simulink model "SPM_trial_2_simulink"  (R2022a)
settings: Solver=VariableStepAuto  StartTime=0.0  StopTime=500  RelTol=1e-3
values from neighbouring files (symbols this model uses):
  x_neg = 0:dx_n:del_n    [Generate_Amat_Electrolyte.m]
  x_pos = del_n+del_s:dx_p:del_n+del_s+del_p    [Generate_Amat_Electrolyte.m]
  x_sep = del_n:dx_s:del_n+del_s    [Generate_Amat_Electrolyte.m]
undefined symbols (not defined in the file or in its folder): CC, cs_init_n, cs_init_p, I, Iin, Ilim, Kaw, KI, nn, np, ns, sw, Vlim, Vmax
libraries: nesl_utility x6, fl_lib x4
settings Model: Creator=YASH PATHAK  LastModifiedBy=YASH PATHAK

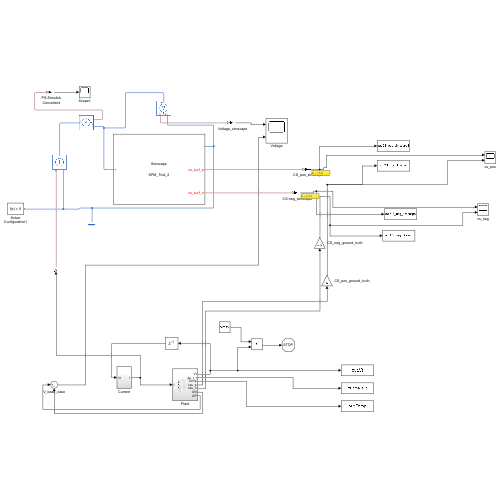
[thumbnail: Simulink's stored preview of the top-level diagram]
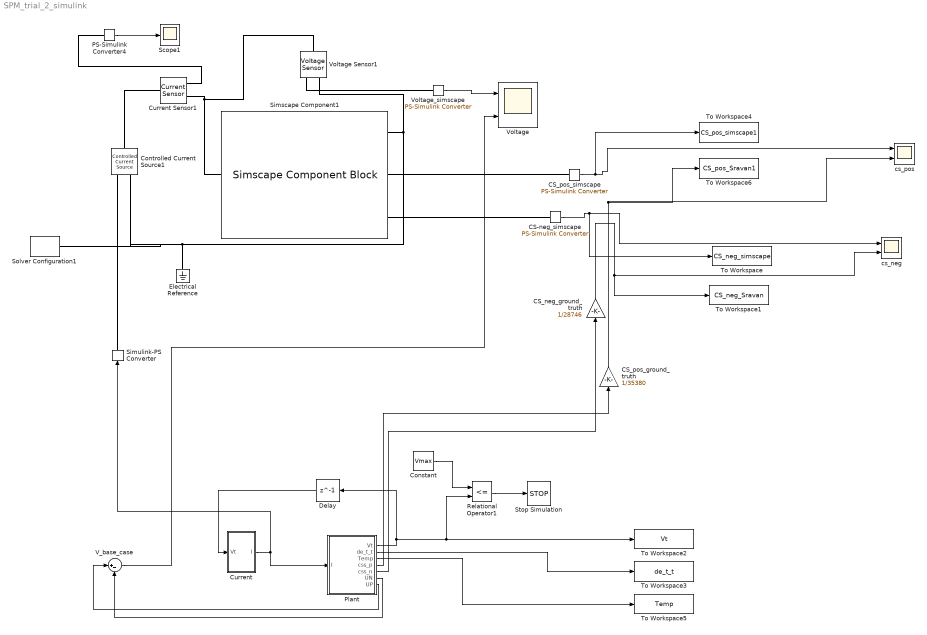
== system SPM_trial_2_simulink ==
  CS-neg_simscape : nesl_utility/PS-Simulink Converter  PhysicalDomain=network_engine_domain  SubClassName=ps_output  LeftPortType=input  RightPortType=output  PseudoPeriodic=off  Frequencies=[]  VectorFormat=inherit  Unit=inherit  AffineConversion=off
      settings: SourceProductBaseCode=SS,PW,VE
  CS_neg_ground_truth : Gain  Gain=1/28746
  CS_pos_ground_truth : Gain  Gain=1/35380
  CS_pos_simscape : nesl_utility/PS-Simulink Converter  PhysicalDomain=network_engine_domain  SubClassName=ps_output  LeftPortType=input  RightPortType=output  PseudoPeriodic=off  Frequencies=[]  VectorFormat=inherit  Unit=inherit  AffineConversion=off
      settings: SourceProductBaseCode=SS,PW,VE
  Constant : Constant  Value=Vmax
  Controlled Current Source1 : fl_lib/Electrical/Electrical Sources/Controlled Current Source
      settings: SourceProductBaseCode=PW,SS,VE
  Current : Subsystem
  Current Sensor1 : fl_lib/Electrical/Electrical Sensors/Current Sensor
      settings: SourceProductBaseCode=PW,SS,VE
  Delay : Delay  DelayLength=1
  Electrical Reference : fl_lib/Electrical/Electrical Elements/Electrical Reference
      settings: SourceProductBaseCode=PW,SS,VE
  PS-Simulink Converter4 : nesl_utility/PS-Simulink Converter  PhysicalDomain=network_engine_domain  SubClassName=ps_output  LeftPortType=input  RightPortType=output  PseudoPeriodic=off  Frequencies=[]  VectorFormat=inherit  Unit=inherit  AffineConversion=off
      settings: SourceProductBaseCode=SS,PW,VE
  Plant : Subsystem
  Relational Operator1 : RelationalOperator  Operator=<=  OutDataTypeStr=boolean  RndMeth=Simplest  InputSameDT=off
  Scope1 : Scope
  Simscape Component1 : SimscapeComponentBlock  SourceFile=SPM_Trial_2  ComponentPath=SPM_Trial_2  ComponentVariants="[\"SPM_Trial_2\"]"  ComponentVariantNames="[\"SPM_Trial_2\"]"  ClassName=SPM_Trial_2  SchemaVersion=1  nr=10  Rp=3.5e-06 m  Rn=2.5e-06 m  Ds_p=8e-15 m^2/s  Ds_n=5e-15 m^2/s  SOC_0=0.1  x100_percent_n=0.8292  x0_percent_n=3.5506e-04  y0_percent_p=0.8941  y100_percent_p=0.0335  del_p=6.7e-05 m  del_n=6.2e-05 m  cs_max_p=35380 mol/m^3  cs_max_n=28746 mol/m^3  epsilon_e_p=0.3  epsilon_e_n=0.3  Active_Area=0.205 m^2  Faradays=96485 C/mol  T=273.15 + 25  R=8.3145  Cap_n=6.0272 C  Cap_p=5.8050 C  i_specify=off  i_priority=None  i=0 A  i_nominal_specify=off  i_nominal_unit=A  i_nominal_value=1  v_specify=off  v_priority=None  v=0 V  v_nominal_specify=off  v_nominal_unit=V  v_nominal_value=1  UP_specify=off  UP_priority=None  UP=0  UP_nominal_specify=off  UP_nominal_unit=1  UP_nominal_value=1  UN_specify=off  UN_priority=None  UN=0  UN_nominal_specify=off  UN_nominal_unit=1  UN_nominal_value=1  V_ocp_specify=off  V_ocp_priority=None  V_ocp=0  V_ocp_nominal_specify=off  V_ocp_nominal_unit=1  V_ocp_nominal_value=1
      settings: CopyFcn=simscape.engine.sli.internal.componentblockcallback(gcbh,'COPY')  PreCopyFcn=simscape.engine.sli.internal.componentblockcallback(gcbh,'PRECOPY')  PreDeleteFcn=simscape.engine.sli.internal.componentblockcallback(gcbh,'PREDELETE')  InternalSimscapePortConfiguration="{\"Bottom\":[],\"Left\":[{\"id\":\"p\",\"label\":\"+\",\"type\":\"foundation.electrical.electrical\"}],\"Right\":[{\"id\":\"n\",\"label\":\"-\",\"type\":\"foundation.electrical.electrical\"},{\"id\":\"cs_surf_p\",\"label\":\"cs_surf_p\",\"type\":\"output\"},{\"id\":\"cs_surf_n\",\"label\":\"cs_surf_n\",\"type\":\"output\"}],\"Top\":[]}"
      mask Type: Two-port electrical component
  Simulink-PS Converter : nesl_utility/Simulink-PS Converter  PhysicalDomain=network_engine_domain  SubClassName=ps_input  LeftPortType=input  RightPortType=output  PseudoPeriodic=off  Frequencies=[]  NoiseDistribution=none  NoiseParameters=[]  Unit=1  AffineConversion=off  FilteringAndDerivatives=provide  SimscapeFilterOrder=1  InputFilterTimeConstant=0.001  UdotUserProvided=0
      settings: SourceProductBaseCode=SS,PW,VE
  Solver Configuration1 : nesl_utility/Solver Configuration  PhysicalDomain=network_engine_domain  SubClassName=solver  LeftPortType=input  RightPortType=generic  Tones=[]  Harmonics=[]  SimulateNoise=off  Profile=off  UseLocalSampling=off  EnableSwitchedLinearOptims=on  FrequencyDomain=off  UseCCode=off  RelTol=0.001  AbsTol=1e-06  MinStep=1e-09  ToWorkspace=off  RevertToSquareIcSolve=off  NumHomotopyIterations=100  PhasorMode=off  PhasorModeNumHarmonics=1  IndexReductionMethod=DerivativeReplacement  DoDC=off  ResidualTolerance=1e-09  UseLocalSolver=off  LocalSolverChoice=NE_BACKWARD_EULER_ADVANCER  LocalSolverSampleTime=0.001  DoFixedCost=off  MaxNonlinIter=3  MaxModeIter=2  ComputeImpulses=off  ImpulseIterations=2  LinearAlgebra=auto  LinearAlgebraNumThread=0  EquationFormulation=NE_TIME_EF  DelaysMemoryBudget=1024  AutomaticFiltering=on  FilteringTimeConstant=0.001  PartitionStorageMethod=AS_NEEDED  PartitionMemoryBudget=1024  PartitionMethod=ROBUST
      settings: SourceProductBaseCode=SS,PW,VE
  Stop Simulation : Stop
  To Workspace : ToWorkspace  VariableName=CS_neg_simscape  SampleTime=-1
  To Workspace1 : ToWorkspace  VariableName=CS_neg_Sravan  SampleTime=-1
  To Workspace2 : ToWorkspace  VariableName=Vt  SampleTime=1
  To Workspace3 : ToWorkspace  VariableName=de_t_t  SampleTime=1
  To Workspace4 : ToWorkspace  VariableName=CS_pos_simscape1  SampleTime=-1
  To Workspace5 : ToWorkspace  VariableName=Temp  SampleTime=1
  To Workspace6 : ToWorkspace  VariableName=CS_pos_Sravan1  SampleTime=-1
  V_base_case : Sum  Inputs=|+-
  Voltage : Scope  NumInputPorts=2
  Voltage Sensor1 : fl_lib/Electrical/Electrical Sensors/Voltage Sensor
      settings: SourceProductBaseCode=PW,SS,VE
  Voltage_simscape : nesl_utility/PS-Simulink Converter  PhysicalDomain=network_engine_domain  SubClassName=ps_output  LeftPortType=input  RightPortType=output  PseudoPeriodic=off  Frequencies=[]  VectorFormat=inherit  Unit=inherit  AffineConversion=off
      settings: SourceProductBaseCode=SS,PW,VE
  cs_neg : Scope  NumInputPorts=2
  cs_pos : Scope  NumInputPorts=2
  wires:
  CS_pos_simscape/1 -> To Workspace4/1, cs_pos/1
  Voltage_simscape/1 -> Voltage/1
  PS-Simulink Converter4/1 -> Scope1/1
  CS-neg_simscape/1 -> To Workspace/1, cs_neg/1
  Current/1(I) -> Plant/1(I), Simulink-PS Converter/1
  Delay/1 -> Current/1(Vt)
  Constant/1 -> Relational Operator1/1
  Relational Operator1/1 -> Stop Simulation/1
  Plant/1(Vt) -> Delay/1, Relational Operator1/2, To Workspace2/1
  Plant/3(Temp) -> To Workspace5/1
  Plant/2(de_t_t) -> To Workspace3/1
  Plant/4(css_p) -> CS_pos_ground_truth/1
  Plant/5(css_n) -> CS_neg_ground_truth/1
  CS_neg_ground_truth/1 -> cs_neg/2, To Workspace1/1
  CS_pos_ground_truth/1 -> To Workspace6/1, cs_pos/2
  Plant/7(UP) -> V_base_case/1
  Plant/6(UN) -> V_base_case/2
  V_base_case/1 -> Voltage/2
  connections:
  Current Sensor1/RConn2 -- Voltage Sensor1/LConn1 -- Simscape Component1/LConn1
  Simscape Component1/RConn1 -- Controlled Current Source1/RConn2 -- Solver Configuration1/RConn1 -- Electrical Reference/LConn1 -- Voltage Sensor1/RConn2
  Voltage Sensor1/RConn1 -- Voltage_simscape/LConn1
  Current Sensor1/RConn1 -- PS-Simulink Converter4/LConn1
  Simscape Component1/RConn2 -- CS_pos_simscape/LConn1
  Simscape Component1/RConn3 -- CS-neg_simscape/LConn1
  Controlled Current Source1/LConn1 -- Current Sensor1/LConn1
  Simulink-PS Converter/RConn1 -- Controlled Current Source1/RConn1

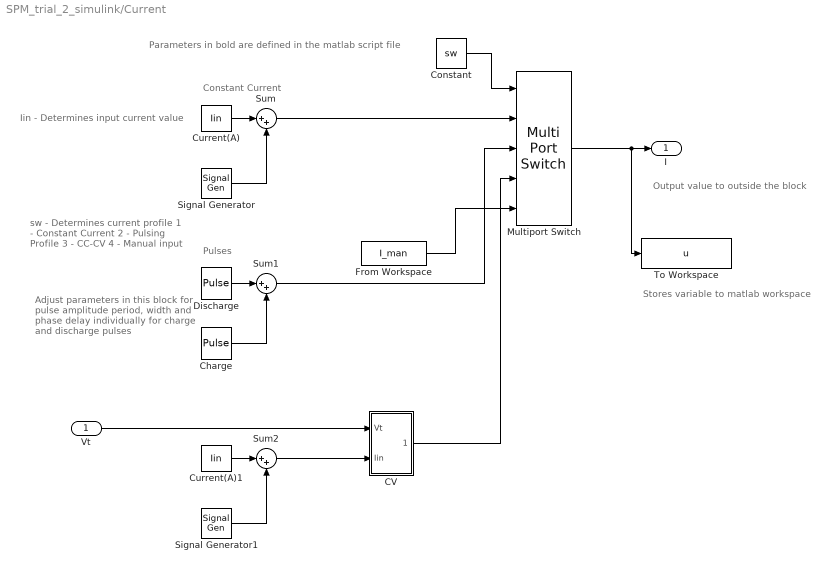
== system SPM_trial_2_simulink/Current ==
  note: Parameters in bold are defined in the matlab script file
  note: Adjust parameters in this block
      | for pulse amplitude period, width
      | and phase delay individually for
      | charge and discharge pulses
  note: Iin - Determines input current value
  note: Constant Current
  note: Pulses
  note: sw - Determines current profile
      | 1 - Constant Current
      | 2 - Pulsing Profile
      | 3 - CC-CV
      | 4 - Manual input
  note: Stores variable to matlab workspace
  note: Output value to outside the block
  Vt : Inport
  CV : Subsystem
  Charge : DiscretePulseGenerator  PulseType=Time based  Amplitude=-Iin/5  Period=100  PulseWidth=25  PhaseDelay=75
  Constant : Constant  Value=sw
  Current(A) : Constant  Value=Iin
  Current(A)1 : Constant  Value=Iin
  Discharge : DiscretePulseGenerator  PulseType=Time based  Amplitude=Iin  Period=100  PulseWidth=25  PhaseDelay=25
  From Workspace : FromWorkspace  VariableName=I_man
  Multiport Switch : MultiPortSwitch  Inputs=4  SaturateOnIntegerOverflow=off  InputSameDT=off
  Signal Generator : SignalGenerator  WaveForm=square  Amplitude=0
  Signal Generator1 : SignalGenerator  WaveForm=square  Amplitude=0  Frequency=0.1
  Sum : Sum  Inputs=|++
  Sum1 : Sum  Inputs=|++
  Sum2 : Sum  Inputs=|++
  To Workspace : ToWorkspace  VariableName=u  SampleTime=1
  I : Outport
  wires:
  Current(A)/1 -> Sum/1
  Discharge/1 -> Sum1/1
  Charge/1 -> Sum1/2
  Signal Generator/1 -> Sum/2
  Sum1/1 -> Multiport Switch/3
  Multiport Switch/1 -> To Workspace/1, I/1
  Sum/1 -> Multiport Switch/2
  Constant/1 -> Multiport Switch/1
  From Workspace/1 -> Multiport Switch/5
  Current(A)1/1 -> Sum2/1
  Sum2/1 -> CV/2(Iin)
  Signal Generator1/1 -> Sum2/2
  Vt/1 -> CV/1(Vt)
  CV/1(Iout) -> Multiport Switch/4

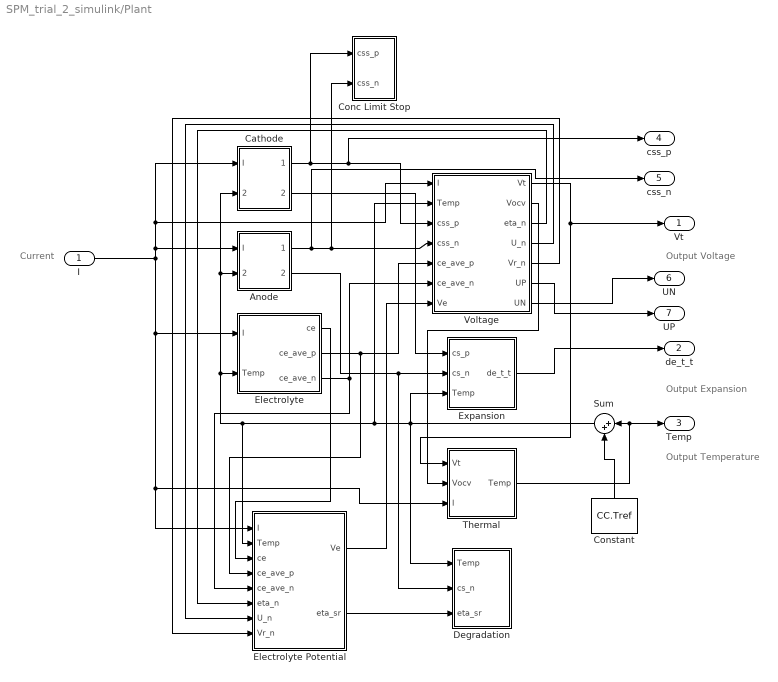
== system SPM_trial_2_simulink/Plant ==
  note: Output Voltage
  note: Output Expansion
  note: Output Temperature
  note: Current
  I : Inport
  Anode : Subsystem
  Cathode : Subsystem
  Conc Limit Stop : Subsystem
  Constant : Constant  Value=CC.Tref
  Degradation : Subsystem
  Electrolyte : Subsystem
  Electrolyte Potential : Subsystem
  Expansion : Subsystem
  Sum : Sum  Inputs=|++
  Thermal : Subsystem
  Voltage : Subsystem
  Vt : Outport
  de_t_t : Outport  Port=2
  Temp : Outport  Port=3
  css_p : Outport  Port=4
  css_n : Outport  Port=5
  UN : Outport  Port=6
  UP : Outport  Port=7
  wires:
  Cathode/2(cs_p) -> Expansion/1(cs_p)
  I/1 -> Cathode/1(I), Voltage/1(I), Anode/1(I), Electrolyte Potential/1(I), Thermal/3(I), Electrolyte/1(I)
  Anode/2(cs_n) -> Degradation/2(cs_n), Expansion/2(cs_n)
  Cathode/1(css_p) -> css_p/1, Voltage/3(css_p), Conc Limit Stop/1(css_p)
  Anode/1(css_n) -> css_n/1, Conc Limit Stop/2(css_n), Voltage/4(css_n)
  Voltage/1(Vt) -> Vt/1, Thermal/1(Vt)
  Sum/1 -> Degradation/1(Temp), Expansion/3(Temp), Voltage/2(Temp), Electrolyte/2(Temp), Cathode/2(Temp), Anode/2(Temp), Electrolyte Potential/2(Temp)
  Expansion/1(de_t_t) -> de_t_t/1
  Electrolyte/2(ce_ave_p) -> Electrolyte Potential/4(ce_ave_p), Voltage/5(ce_ave_p)
  Electrolyte/3(ce_ave_n) -> Electrolyte Potential/5(ce_ave_n), Voltage/6(ce_ave_n)
  Voltage/2(Vocv) -> Thermal/2(Vocv)
  Electrolyte/1(ce) -> Electrolyte Potential/3(ce)
  Voltage/3(eta_n) -> Electrolyte Potential/6(eta_n)
  Voltage/4(U_n) -> Electrolyte Potential/7(U_n)
  Voltage/5(Vr_n) -> Electrolyte Potential/8(Vr_n)
  Electrolyte Potential/1(Ve) -> Voltage/7(Ve)
  Electrolyte Potential/2(eta_sr) -> Degradation/3(eta_sr)
  Thermal/1(Temp) -> Temp/1, Sum/1
  Constant/1 -> Sum/2
  Voltage/7(UN) -> UN/1
  Voltage/6(UP) -> UP/1

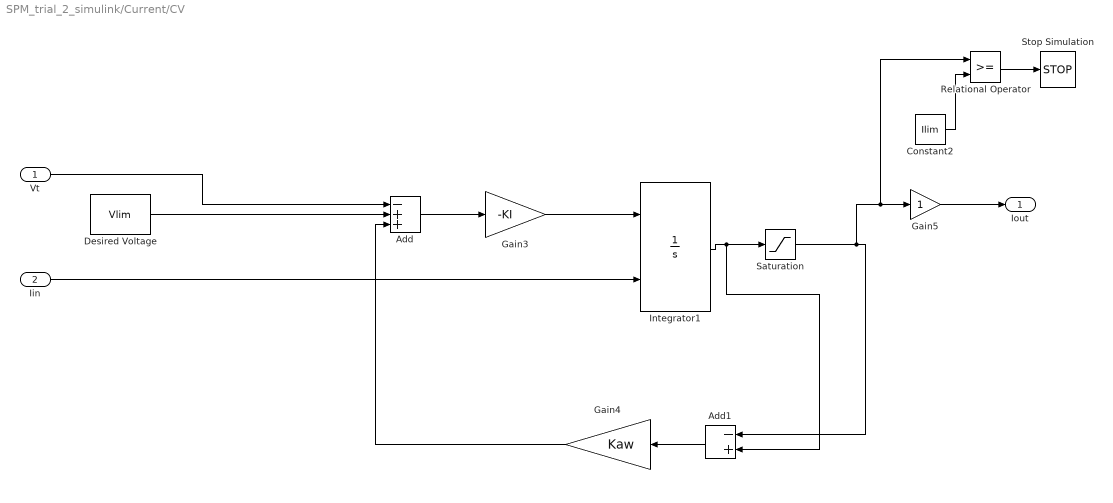
== system SPM_trial_2_simulink/Current/CV ==
  Vt : Inport
  Iin : Inport  Port=2
  Add : Sum  Inputs=-++
  Add1 : Sum  Inputs=-+
  Constant2 : Constant  Value=Ilim
  Desired Voltage : Constant  Value=Vlim
  Gain3 : Gain  Gain=-KI
  Gain4 : Gain  Gain=Kaw
  Gain5 : Gain
  Integrator1 : Integrator  InitialConditionSource=external  InitialCondition=I  UpperSaturationLimit=0  LowerSaturationLimit=-4.5
  Relational Operator : RelationalOperator  OutDataTypeStr=boolean  RndMeth=Simplest  InputSameDT=off
  Saturation : Saturate  UpperLimit=inf  LowerLimit=Iin
  Stop Simulation : Stop
  Iout : Outport
  wires:
  Vt/1 -> Add/1
  Iin/1 -> Integrator1/2
  Add/1 -> Gain3/1
  Add1/1 -> Gain4/1
  Gain4/1 -> Add/3
  Desired Voltage/1 -> Add/2
  Gain3/1 -> Integrator1/1
  Integrator1/1 -> Add1/2, Saturation/1
  Gain5/1 -> Iout/1
  Saturation/1 -> Relational Operator/1, Gain5/1, Add1/1
  Constant2/1 -> Relational Operator/2
  Relational Operator/1 -> Stop Simulation/1

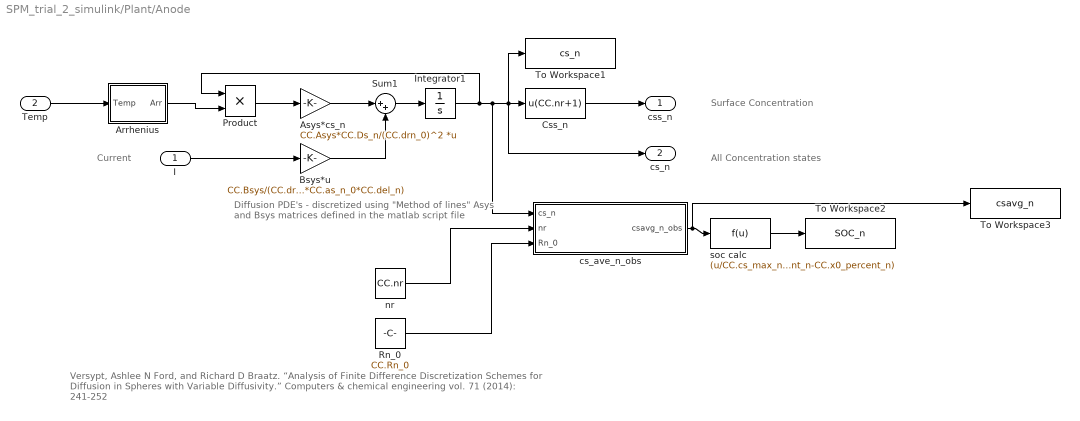
== system SPM_trial_2_simulink/Plant/Anode ==
  note: Current
  note: Surface Concentration
  note: All Concentration states
  note: Diffusion PDE's - discretized using "Method of lines"
      | Asys and Bsys matrices defined in the matlab script file
  note: Versypt, Ashlee N Ford, and Richard D Braatz. “Analysis of Finite Difference Discretization Schemes for Diffusion in Spheres with Variable Diffusivity.” Computers & chemical engineering vol. 71 (2014): 241-252
  I : Inport
  Temp : Inport  Port=2
  Arrhenius : Subsystem
  Asys*cs_n : Gain  Gain=CC.Asys*CC.Ds_n/(CC.drn_0)^2  Multiplication=Matrix(K*u)
  Bsys*u : Gain  Gain=CC.Bsys/(CC.drn_0*CC.F*CC.A*CC.as_n_0*CC.del_n)
  Css_n : Fcn  Expr=u(CC.nr+1)
  Integrator1 : Integrator  InitialCondition=cs_init_n*ones(CC.nr+1,1)
  Product : Product
  Rn_0 : Constant  Value=CC.Rn_0
  Sum1 : Sum  Inputs=|++
  To Workspace1 : ToWorkspace  VariableName=cs_n  SampleTime=1
  To Workspace2 : ToWorkspace  VariableName=SOC_n  SampleTime=1
  To Workspace3 : ToWorkspace  VariableName=csavg_n  SampleTime=1
  cs_ave_n_obs : MATLAB Function  TreatAsAtomicUnit=on
  nr : Constant  Value=CC.nr
  soc calc : Fcn  Expr=(u/CC.cs_max_n-CC.x0_percent_n)/(CC.x100_percent_n-CC.x0_percent_n)
  css_n : Outport
  cs_n : Outport  Port=2
  wires:
  Integrator1/1 -> Product/1, cs_ave_n_obs/1(cs_n), cs_n/1, Css_n/1, To Workspace1/1
  Asys*cs_n/1 -> Sum1/1
  Bsys*u/1 -> Sum1/2
  I/1 -> Bsys*u/1
  Sum1/1 -> Integrator1/1
  Css_n/1 -> css_n/1
  Rn_0/1 -> cs_ave_n_obs/3(Rn_0)
  nr/1 -> cs_ave_n_obs/2(nr)
  cs_ave_n_obs/1(csavg_n_obs) -> To Workspace3/1, soc calc/1
  soc calc/1 -> To Workspace2/1
  Arrhenius/1(Arr) -> Product/2
  Temp/1 -> Arrhenius/1(Temp)
  Product/1 -> Asys*cs_n/1

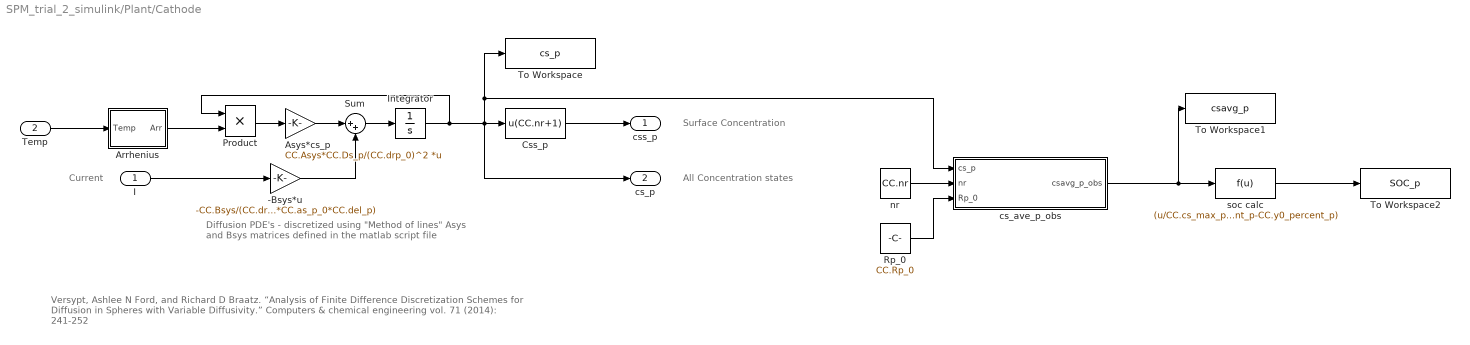
== system SPM_trial_2_simulink/Plant/Cathode ==
  note: Diffusion PDE's - discretized using "Method of lines"
      | Asys and Bsys matrices defined in the matlab script file
  note: All Concentration states
  note: Surface Concentration
  note: Current
  note: Versypt, Ashlee N Ford, and Richard D Braatz. “Analysis of Finite Difference Discretization Schemes for Diffusion in Spheres with Variable Diffusivity.” Computers & chemical engineering vol. 71 (2014): 241-252
  I : Inport
  Temp : Inport  Port=2
  -Bsys*u : Gain  Gain=-CC.Bsys/(CC.drp_0*CC.F*CC.A*CC.as_p_0*CC.del_p)
  Arrhenius : Subsystem
  Asys*cs_p : Gain  Gain=CC.Asys*CC.Ds_p/(CC.drp_0)^2  Multiplication=Matrix(K*u)
  Css_p : Fcn  Expr=u(CC.nr+1)
  Integrator : Integrator  InitialCondition=cs_init_p*ones(CC.nr+1,1)
  Product : Product
  Rp_0 : Constant  Value=CC.Rp_0
  Sum : Sum  Inputs=|++
  To Workspace : ToWorkspace  VariableName=cs_p  SampleTime=1
  To Workspace1 : ToWorkspace  VariableName=csavg_p  SampleTime=1
  To Workspace2 : ToWorkspace  VariableName=SOC_p  SampleTime=1
  cs_ave_p_obs : MATLAB Function  TreatAsAtomicUnit=on
  nr : Constant  Value=CC.nr
  soc calc : Fcn  Expr=(u/CC.cs_max_p-CC.y0_percent_p)/(CC.y100_percent_p-CC.y0_percent_p)
  css_p : Outport
  cs_p : Outport  Port=2
  wires:
  Arrhenius/1(Arr) -> Product/2
  Temp/1 -> Arrhenius/1(Temp)
  Product/1 -> Asys*cs_p/1
  Rp_0/1 -> cs_ave_p_obs/3(Rp_0)
  cs_ave_p_obs/1(csavg_p_obs) -> soc calc/1, To Workspace1/1
  Integrator/1 -> To Workspace/1, cs_ave_p_obs/1(cs_p), Css_p/1, cs_p/1, Product/1
  nr/1 -> cs_ave_p_obs/2(nr)
  soc calc/1 -> To Workspace2/1
  I/1 -> -Bsys*u/1
  Css_p/1 -> css_p/1
  Asys*cs_p/1 -> Sum/1
  Sum/1 -> Integrator/1
  -Bsys*u/1 -> Sum/2

== system SPM_trial_2_simulink/Plant/Conc Limit Stop ==
  css_p : Inport
  css_n : Inport  Port=2
  Constant1 : Constant  Value=0
  Constant2 : Constant  Value=CC.cs_max_p
  Constant3 : Constant  Value=0
  Constant4 : Constant  Value=CC.cs_max_n
  OR : Logic  Operator=OR  Inputs=4  IconShape=distinctive  AllPortsSameDT=off  OutDataTypeStr=boolean
  Relational Operator1 : RelationalOperator  Operator=<=  OutDataTypeStr=boolean  RndMeth=Simplest  InputSameDT=off
  Relational Operator2 : RelationalOperator  Operator=<=  OutDataTypeStr=boolean  RndMeth=Simplest  InputSameDT=off
  Relational Operator3 : RelationalOperator  OutDataTypeStr=boolean  RndMeth=Simplest  InputSameDT=off
  Relational Operator4 : RelationalOperator  OutDataTypeStr=boolean  RndMeth=Simplest  InputSameDT=off
  Stop Simulation1 : Stop
  wires:
  Constant3/1 -> Relational Operator3/1
  Relational Operator3/1 -> OR/3
  Relational Operator2/1 -> OR/4
  css_n/1 -> Relational Operator2/2, Relational Operator3/2
  Constant4/1 -> Relational Operator2/1
  Constant2/1 -> Relational Operator1/1
  Constant1/1 -> Relational Operator4/1
  OR/1 -> Stop Simulation1/1
  Relational Operator1/1 -> OR/2
  css_p/1 -> Relational Operator1/2, Relational Operator4/2
  Relational Operator4/1 -> OR/1

== system SPM_trial_2_simulink/Plant/Degradation ==
  Temp : Inport
  cs_n : Inport  Port=2
  eta_sr : Inport  Port=3
  Mechanical Stress : Subsystem
  Plating : Subsystem
  SEI : Subsystem
  wires:
  Temp/1 -> SEI/2(Temp), Plating/2(Temp)
  eta_sr/1 -> Plating/1(eta_sr), SEI/1(eta_sr)
  cs_n/1 -> Mechanical Stress/1(cs_n)

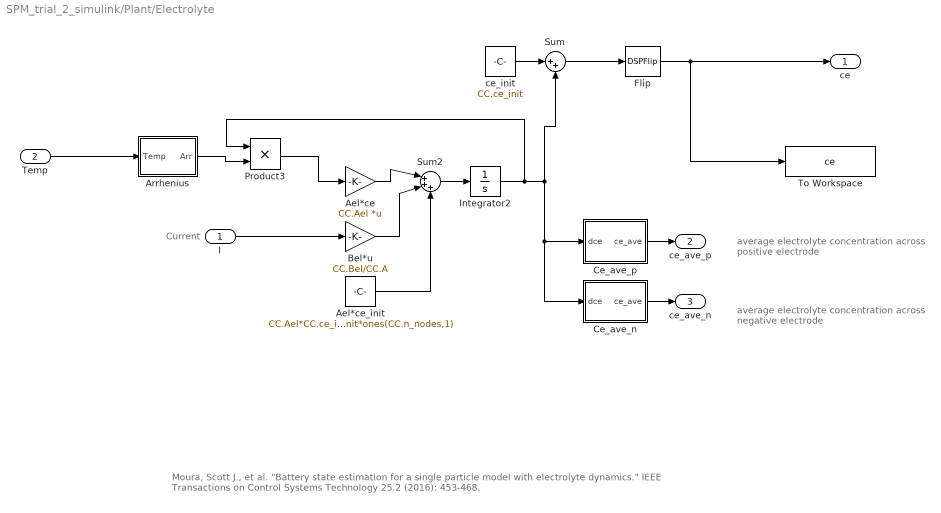
== system SPM_trial_2_simulink/Plant/Electrolyte ==
  note: Moura, Scott J., et al. "Battery state estimation for a single particle model with electrolyte dynamics." IEEE Transactions on Control Systems Technology 25.2 (2016): 453-468.
  note: Current
  note: average electrolyte concentration across
      | negative electrode
  note: average electrolyte concentration across
      | positive electrode
  I : Inport
  Temp : Inport  Port=2
  Ael*ce : Gain  Gain=CC.Ael  Multiplication=Matrix(K*u)
  Ael*ce_init : Constant  Value=CC.Ael*CC.ce_init*ones(CC.n_nodes,1)
  Arrhenius : Subsystem
  Bel*u : Gain  Gain=CC.Bel/CC.A
  Ce_ave_n : Subsystem
  Ce_ave_p : Subsystem
  Flip : DSPFlip
  Integrator2 : Integrator  InitialCondition=zeros(CC.n_nodes,1)
  Product3 : Product
  Sum : Sum  Inputs=|++
  Sum2 : Sum  Inputs=|+++
  To Workspace : ToWorkspace  VariableName=ce  SampleTime=1
  ce_init : Constant  Value=CC.ce_init
  ce : Outport
  ce_ave_p : Outport  Port=2
  ce_ave_n : Outport  Port=3
  wires:
  Temp/1 -> Arrhenius/1(Temp)
  Product3/1 -> Ael*ce/1
  Arrhenius/1(Arr) -> Product3/2
  Flip/1 -> To Workspace/1, ce/1
  I/1 -> Bel*u/1
  Ce_ave_n/1(ce_ave) -> ce_ave_n/1
  ce_init/1 -> Sum/1
  Sum/1 -> Flip/1
  Ce_ave_p/1(ce_ave) -> ce_ave_p/1
  Ael*ce/1 -> Sum2/1
  Bel*u/1 -> Sum2/2
  Sum2/1 -> Integrator2/1
  Ael*ce_init/1 -> Sum2/3
  Integrator2/1 -> Ce_ave_p/1(dce), Ce_ave_n/1(dce), Sum/2, Product3/1

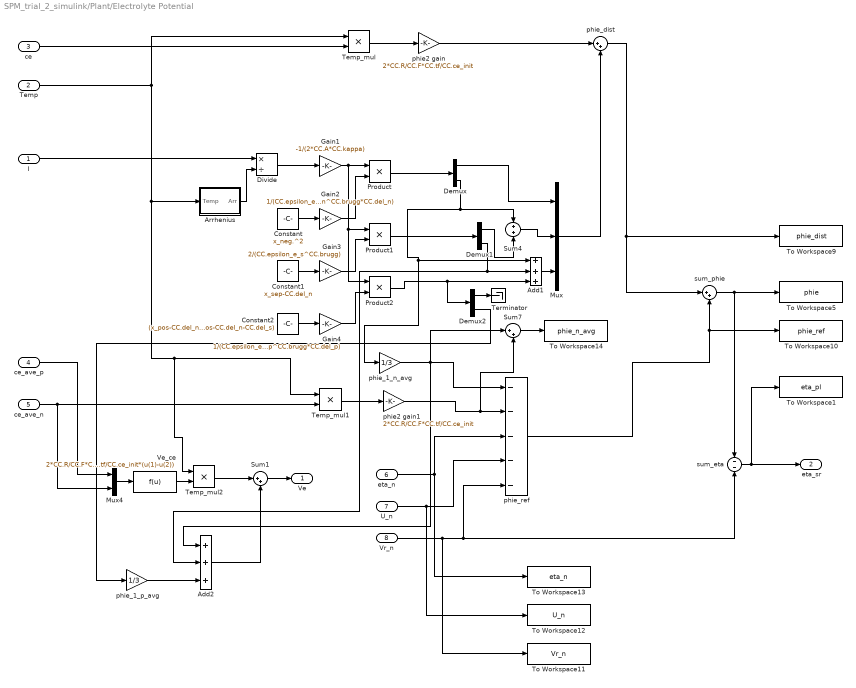
== system SPM_trial_2_simulink/Plant/Electrolyte Potential ==
  I : Inport
  Temp : Inport  Port=2
  ce : Inport  Port=3
  ce_ave_p : Inport  Port=4
  ce_ave_n : Inport  Port=5
  eta_n : Inport  Port=6
  U_n : Inport  Port=7
  Vr_n : Inport  Port=8
  Add1 : Sum  Inputs=+++
  Add2 : Sum  Inputs=+++
  Arrhenius : Subsystem
  Constant : Constant  Value=x_neg.^2
  Constant1 : Constant  Value=x_sep-CC.del_n
  Constant2 : Constant  Value=(x_pos-CC.del_n-CC.del_s).*(2*CC.del_t-x_pos-CC.del_n-CC.del_s)
  Demux : Demux  Outputs=[nn,1]
  Demux1 : Demux  Outputs=[ns,1]
  Demux2 : Demux  Outputs=[np,1]
  Divide : Product  Inputs=*/
  Gain1 : Gain  Gain=-1/(2*CC.A*CC.kappa)
  Gain2 : Gain  Gain=1/(CC.epsilon_e_n^CC.brugg*CC.del_n)
  Gain3 : Gain  Gain=2/(CC.epsilon_e_s^CC.brugg)
  Gain4 : Gain  Gain=1/(CC.epsilon_e_p^CC.brugg*CC.del_p)
  Mux : Mux  Inputs=3
  Mux4 : Mux  Inputs=2
  Product : Product
  Product1 : Product
  Product2 : Product
  Sum1 : Sum  Inputs=|++
  Sum4 : Sum
  Sum7 : Sum  Inputs=|++
  Temp_mul : Product
  Temp_mul1 : Product
  Temp_mul2 : Product
  Terminator : Terminator
  To Workspace1 : ToWorkspace  VariableName=eta_pl  SampleTime=1
  To Workspace10 : ToWorkspace  VariableName=phie_ref  SampleTime=1
  To Workspace11 : ToWorkspace  VariableName=Vr_n  SampleTime=1
  To Workspace12 : ToWorkspace  VariableName=U_n  SampleTime=1
  To Workspace13 : ToWorkspace  VariableName=eta_n  SampleTime=1
  To Workspace14 : ToWorkspace  VariableName=phie_n_avg  SampleTime=1
  To Workspace5 : ToWorkspace  VariableName=phie  SampleTime=1
  To Workspace9 : ToWorkspace  VariableName=phie_dist  SampleTime=1
  Ve_ce : Fcn  Expr=2*CC.R/CC.F*CC.tf/CC.ce_init*(u(1)-u(2))
  phie2 gain : Gain  Gain=2*CC.R/CC.F*CC.tf/CC.ce_init
  phie2 gain1 : Gain  Gain=2*CC.R/CC.F*CC.tf/CC.ce_init
  phie_1_n_avg : Gain  Gain=1/3
  phie_1_p_avg : Gain  Gain=1/3
  phie_dist : Sum  Inputs=|++
  phie_ref : Sum  Inputs=-----
  sum_eta : Sum  Inputs=--
  sum_phie : Sum  Inputs=|++
  Ve : Outport
  eta_sr : Outport  Port=2
  wires:
  I/1 -> Divide/1
  ce_ave_n/1 -> Mux4/2, Temp_mul1/2
  ce/1 -> Temp_mul/2
  sum_eta/1 -> eta_sr/1, To Workspace1/1
  phie_ref/1 -> To Workspace10/1, sum_phie/2
  phie_1_n_avg/1 -> Add2/1, Sum7/1, phie_ref/1
  Temp/1 -> Temp_mul/1, Arrhenius/1(Temp), Temp_mul2/1, Temp_mul1/1
  Demux/1 -> Mux/1
  Gain1/1 -> Product2/1, Product1/1, Product/1
  Constant/1 -> Gain2/1
  Arrhenius/1(Arr) -> Divide/2
  Constant1/1 -> Gain3/1
  Gain4/1 -> Product2/2
  Product1/1 -> Demux1/1
  Mux/1 -> phie_dist/2
  Gain3/1 -> Product1/2
  Gain2/1 -> Product/2
  sum_phie/1 -> sum_eta/1, To Workspace5/1
  Temp_mul1/1 -> phie2 gain1/1
  phie2 gain/1 -> phie_dist/1
  Product/1 -> Demux/1
  phie2 gain1/1 -> Sum7/2, phie_ref/2
  Vr_n/1 -> phie_ref/5, sum_eta/2, To Workspace11/1
  Demux/2 -> Sum4/1, Add1/1, phie_1_n_avg/1
  eta_n/1 -> phie_ref/3, To Workspace13/1
  Temp_mul/1 -> phie2 gain/1
  phie_dist/1 -> To Workspace9/1, sum_phie/1
  Constant2/1 -> Gain4/1
  Product2/1 -> Demux2/1, Add1/3
  U_n/1 -> phie_ref/4, To Workspace12/1
  Divide/1 -> Gain1/1
  Sum7/1 -> To Workspace14/1
  Mux4/1 -> Ve_ce/1
  ce_ave_p/1 -> Mux4/1
  Ve_ce/1 -> Temp_mul2/2
  Temp_mul2/1 -> Sum1/1
  Sum4/1 -> Mux/2
  Demux1/1 -> Sum4/2
  Add1/1 -> Mux/3
  Demux1/2 -> Add1/2, Add2/2
  Demux2/1 -> Terminator/1
  phie_1_p_avg/1 -> Add2/3
  Demux2/2 -> phie_1_p_avg/1
  Add2/1 -> Sum1/2
  Sum1/1 -> Ve/1

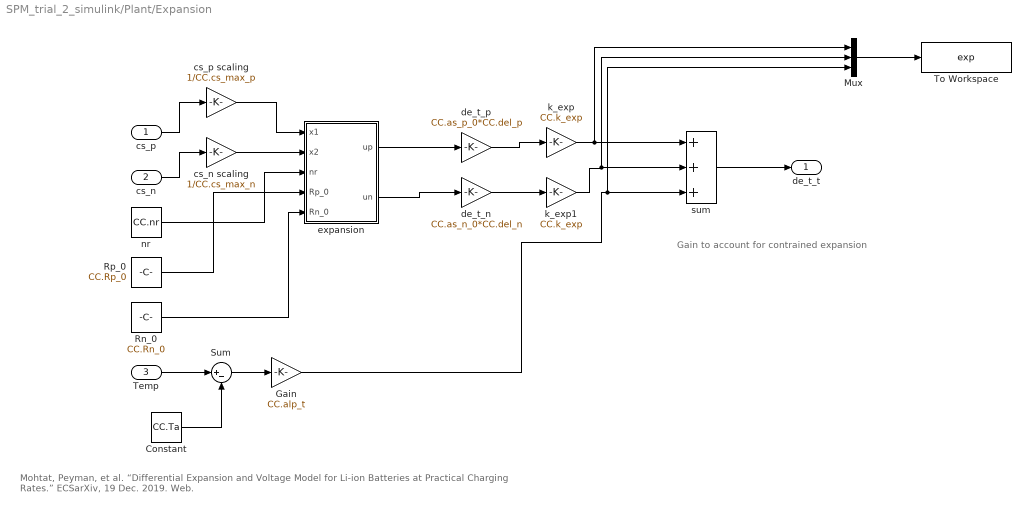
== system SPM_trial_2_simulink/Plant/Expansion ==
  note: Gain to account for contrained expansion
  note: Mohtat, Peyman, et al. “Differential Expansion and Voltage Model for Li-ion Batteries at Practical Charging Rates.” ECSarXiv, 19 Dec. 2019. Web.
  cs_p : Inport
  cs_n : Inport  Port=2
  Temp : Inport  Port=3
  Constant : Constant  Value=CC.Ta
  Gain : Gain  Gain=CC.alp_t
  Mux : Mux  Inputs=3
  Rn_0 : Constant  Value=CC.Rn_0
  Rp_0 : Constant  Value=CC.Rp_0
  Sum : Sum  Inputs=|+-
  To Workspace : ToWorkspace  VariableName=exp  SampleTime=1
  cs_n scaling : Gain  Gain=1/CC.cs_max_n
  cs_p scaling : Gain  Gain=1/CC.cs_max_p
  de_t_n : Gain  Gain=CC.as_n_0*CC.del_n
  de_t_p : Gain  Gain=CC.as_p_0*CC.del_p
  expansion : MATLAB Function  TreatAsAtomicUnit=on
  k_exp : Gain  Gain=CC.k_exp
  k_exp1 : Gain  Gain=CC.k_exp
  nr : Constant  Value=CC.nr
  sum : Sum  Inputs=+++
  de_t_t : Outport
  wires:
  de_t_n/1 -> k_exp1/1
  cs_n/1 -> cs_n scaling/1
  Rp_0/1 -> expansion/4(Rp_0)
  Rn_0/1 -> expansion/5(Rn_0)
  nr/1 -> expansion/3(nr)
  de_t_p/1 -> k_exp/1
  cs_p/1 -> cs_p scaling/1
  expansion/1(up) -> de_t_p/1
  expansion/2(un) -> de_t_n/1
  cs_p scaling/1 -> expansion/1(x1)
  cs_n scaling/1 -> expansion/2(x2)
  Temp/1 -> Sum/1
  Constant/1 -> Sum/2
  Sum/1 -> Gain/1
  Gain/1 -> Mux/3, sum/3
  sum/1 -> de_t_t/1
  Mux/1 -> To Workspace/1
  k_exp/1 -> Mux/1, sum/1
  k_exp1/1 -> Mux/2, sum/2

== system SPM_trial_2_simulink/Plant/Thermal ==
  note: Note: Ignoring entropic heating
  Vt : Inport
  Vocv : Inport  Port=2
  I : Inport  Port=3
  Abs : Abs  SaturateOnIntegerOverflow=off
  Constant : Constant  Value=CC.Ta
  Convection : Gain  Gain=CC.h
  Integrator : Integrator  InitialCondition=CC.T0
  Product : Product
  Scope : Scope
  Sum : Sum  Inputs=|+-
  Sum1 : Sum  Inputs=|-+
  Sum2 : Sum  Inputs=|+-
  Thermal Mass : Gain  Gain=1/CC.th_mass
  Temp : Outport
  wires:
  Sum1/1 -> Convection/1
  Abs/1 -> Sum2/1
  Integrator/1 -> Scope/1, Temp/1, Sum1/2
  Sum2/1 -> Thermal Mass/1
  Constant/1 -> Sum1/1
  Convection/1 -> Sum2/2
  Vt/1 -> Sum/1
  Vocv/1 -> Sum/2
  Sum/1 -> Product/1
  I/1 -> Product/2
  Product/1 -> Abs/1
  Thermal Mass/1 -> Integrator/1

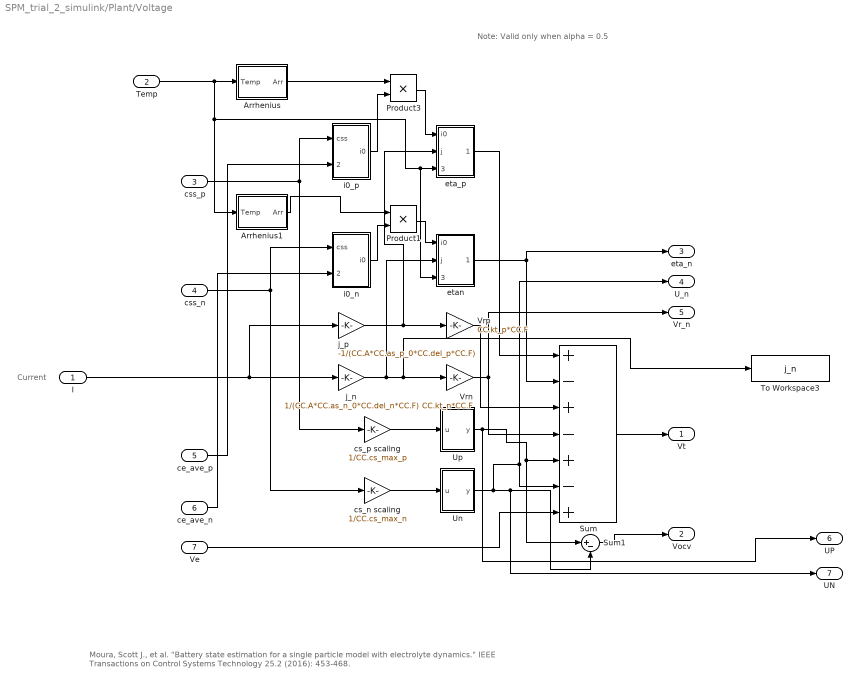
== system SPM_trial_2_simulink/Plant/Voltage ==
  note: Note: Valid only when alpha = 0.5
  note: Current
  note: Moura, Scott J., et al. "Battery state estimation for a single particle model with electrolyte dynamics." IEEE Transactions on Control Systems Technology 25.2 (2016): 453-468.
  I : Inport
  Temp : Inport  Port=2
  css_p : Inport  Port=3
  css_n : Inport  Port=4
  ce_ave_p : Inport  Port=5
  ce_ave_n : Inport  Port=6
  Ve : Inport  Port=7
  Arrhenius : Subsystem
  Arrhenius1 : Subsystem
  Product1 : Product
  Product3 : Product
  Sum : Sum  Inputs=+-+-+-+
  Sum1 : Sum  Inputs=|+-
  To Workspace3 : ToWorkspace  VariableName=j_n  SampleTime=1
  Un : MATLAB Function  TreatAsAtomicUnit=on
  Up : MATLAB Function  TreatAsAtomicUnit=on
  Vrn : Gain  Gain=CC.kt_n*CC.F
  Vrp : Gain  Gain=CC.kt_p*CC.F
  cs_n scaling : Gain  Gain=1/CC.cs_max_n
  cs_p scaling : Gain  Gain=1/CC.cs_max_p
  eta_p : Subsystem
  etan : Subsystem
  i0_n : Subsystem
  i0_p : Subsystem
  j_n : Gain  Gain=1/(CC.A*CC.as_n_0*CC.del_n*CC.F)
  j_p : Gain  Gain=-1/(CC.A*CC.as_p_0*CC.del_p*CC.F)
  Vt : Outport
  Vocv : Outport  Port=2
  eta_n : Outport  Port=3
  U_n : Outport  Port=4
  Vr_n : Outport  Port=5
  UP : Outport  Port=6
  UN : Outport  Port=7
  wires:
  j_n/1 -> etan/2(j), To Workspace3/1, Vrn/1
  j_p/1 -> Vrp/1, eta_p/2(j)
  eta_p/1(eta) -> Sum/1
  etan/1(eta) -> Sum/2, eta_n/1
  cs_n scaling/1 -> Un/1(u)
  i0_p/1(i0) -> Product3/2
  i0_n/1(i0) -> Product1/2
  cs_p scaling/1 -> Up/1(u)
  I/1 -> j_p/1, j_n/1
  css_p/1 -> cs_p scaling/1, i0_p/1(css)
  Up/1(y) -> UP/1, Sum1/1, Sum/5
  css_n/1 -> cs_n scaling/1, i0_n/1(css)
  Un/1(y) -> UN/1, Sum1/2, U_n/1, Sum/6
  Vrp/1 -> Sum/3
  ce_ave_p/1 -> i0_p/2(ce_ave)
  ce_ave_n/1 -> i0_n/2(ce_ave)
  Sum/1 -> Vt/1
  Sum1/1 -> Vocv/1
  Vrn/1 -> Vr_n/1, Sum/4
  Temp/1 -> Arrhenius/1(Temp), Arrhenius1/1(Temp), eta_p/3(Temp), etan/3(Temp)
  Product3/1 -> eta_p/1(i0)
  Arrhenius1/1(Arr) -> Product1/1
  Product1/1 -> etan/1(i0)
  Ve/1 -> Sum/7
  Arrhenius/1(Arr) -> Product3/1

== system SPM_trial_2_simulink/Plant/Anode/Arrhenius ==
  Temp : Inport
  Constant : Constant  Value=1/CC.T
  Gain : Gain  Gain=CC.E_Ds_n/CC.R
  Math Function : Math
  Reciprocal : Product  Inputs=/
  Subtract : Sum  Inputs=+-
  Arr : Outport
  wires:
  Subtract/1 -> Gain/1
  Reciprocal/1 -> Subtract/2
  Constant/1 -> Subtract/1
  Math Function/1 -> Arr/1
  Temp/1 -> Reciprocal/1
  Gain/1 -> Math Function/1

== system SPM_trial_2_simulink/Plant/Cathode/Arrhenius ==
  Temp : Inport
  Constant : Constant  Value=1/CC.T
  Gain : Gain  Gain=CC.E_Ds_p/CC.R
  Math Function : Math
  Reciprocal : Product  Inputs=/
  Subtract : Sum  Inputs=+-
  Arr : Outport
  wires:
  Subtract/1 -> Gain/1
  Reciprocal/1 -> Subtract/2
  Constant/1 -> Subtract/1
  Math Function/1 -> Arr/1
  Temp/1 -> Reciprocal/1
  Gain/1 -> Math Function/1

== system SPM_trial_2_simulink/Plant/Degradation/Mechanical Stress ==
  cs_n : Inport
  Add : Sum
  Gain : Gain  Gain=1/3
  Gain1 : Gain  Gain=2/3
  Rn_1 : Constant  Value=CC.Rn_0
  To Workspace4 : ToWorkspace  VariableName=sigma_r  SampleTime=1
      settings: Save2DSignal=2-D array (concatenate along first dimension)
  To Workspace5 : ToWorkspace  VariableName=sigma_t  SampleTime=1
      settings: Save2DSignal=2-D array (concatenate along first dimension)
  To Workspace6 : ToWorkspace  VariableName=sigma_h  SampleTime=1
      settings: Save2DSignal=2-D array (concatenate along first dimension)
  const : Constant  Value=CC.Omega_nP*CC.E_nP/3/(1-CC.v_nP)
  nr1 : Constant  Value=CC.nr
  sigma : MATLAB Function  TreatAsAtomicUnit=on
  wires:
  sigma/2(sigma_t) -> Gain1/1, To Workspace5/1
  sigma/1(sigma_r) -> Gain/1, To Workspace4/1
  cs_n/1 -> sigma/1(cs_n)
  nr1/1 -> sigma/2(nr)
  Add/1 -> To Workspace6/1
  const/1 -> sigma/4(const)
  Gain/1 -> Add/1
  Gain1/1 -> Add/2
  Rn_1/1 -> sigma/3(Rn_0)

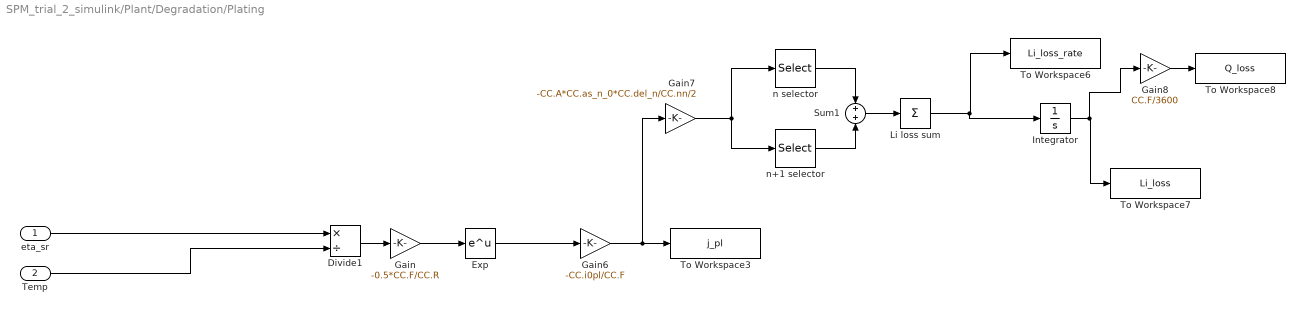
== system SPM_trial_2_simulink/Plant/Degradation/Plating ==
  eta_sr : Inport
  Temp : Inport  Port=2
  Divide1 : Product  Inputs=*/
  Exp : Math
  Gain : Gain  Gain=-0.5*CC.F/CC.R
  Gain6 : Gain  Gain=-CC.i0pl/CC.F
  Gain7 : Gain  Gain=-CC.A*CC.as_n_0*CC.del_n/CC.nn/2
  Gain8 : Gain  Gain=CC.F/3600
  Integrator : Integrator
  Li loss sum : Sum  Inputs=+
  Sum1 : Sum
  To Workspace3 : ToWorkspace  VariableName=j_pl  SampleTime=1
  To Workspace6 : ToWorkspace  VariableName=Li_loss_rate  SampleTime=1
  To Workspace7 : ToWorkspace  VariableName=Li_loss  SampleTime=1
  To Workspace8 : ToWorkspace  VariableName=Q_loss  SampleTime=1
  n selector : Selector  InputPortWidth=CC.n_nodes  IndexOptions=Index vector (dialog)  Indices=[1:CC.nn]  OutputSizes=1
  n+1 selector : Selector  InputPortWidth=CC.n_nodes  IndexOptions=Index vector (dialog)  Indices=[2:CC.nn+1]  OutputSizes=1
  wires:
  Gain6/1 -> Gain7/1, To Workspace3/1
  Gain7/1 -> n selector/1, n+1 selector/1
  Li loss sum/1 -> Integrator/1, To Workspace6/1
  Exp/1 -> Gain6/1
  Divide1/1 -> Gain/1
  Gain/1 -> Exp/1
  Sum1/1 -> Li loss sum/1
  Integrator/1 -> Gain8/1, To Workspace7/1
  Gain8/1 -> To Workspace8/1
  n selector/1 -> Sum1/1
  n+1 selector/1 -> Sum1/2
  eta_sr/1 -> Divide1/1
  Temp/1 -> Divide1/2

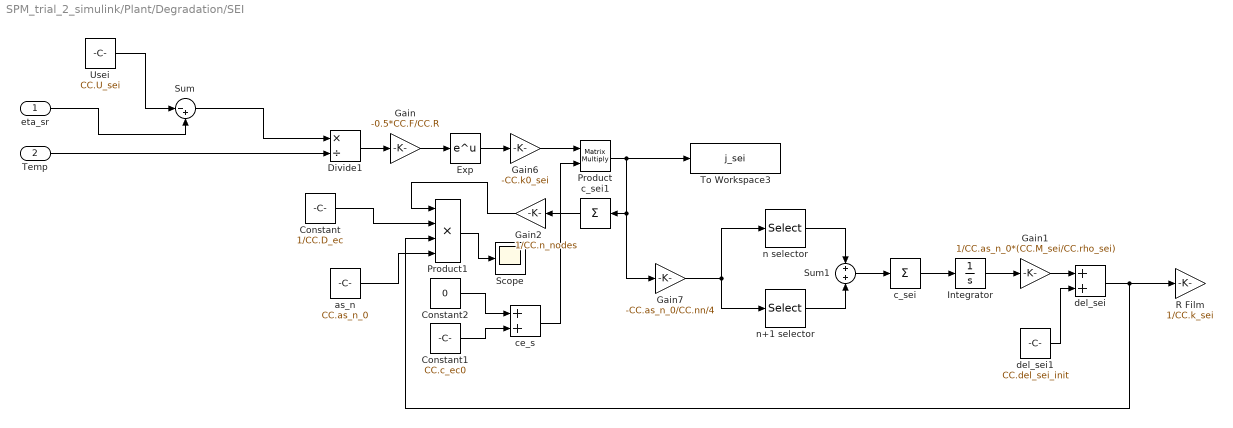
== system SPM_trial_2_simulink/Plant/Degradation/SEI ==
  eta_sr : Inport
  Temp : Inport  Port=2
  Constant : Constant  Value=1/CC.D_ec
  Constant1 : Constant  Value=CC.c_ec0
  Constant2 : Constant  Value=0
  Divide1 : Product  Inputs=*/
  Exp : Math
  Gain : Gain  Gain=-0.5*CC.F/CC.R
  Gain1 : Gain  Gain=1/CC.as_n_0*(CC.M_sei/CC.rho_sei)
  Gain2 : Gain  Gain=1/CC.n_nodes
  Gain6 : Gain  Gain=-CC.k0_sei
  Gain7 : Gain  Gain=-CC.as_n_0/CC.nn/4
  Integrator : Integrator
  Product : Product  Multiplication=Matrix(*)
  Product1 : Product  Inputs=4
  R Film : Gain  Gain=1/CC.k_sei
  Scope : Scope
  Sum : Sum  Inputs=|-+
  Sum1 : Sum
  To Workspace3 : ToWorkspace  VariableName=j_sei  SampleTime=1
  Usei : Constant  Value=CC.U_sei
  as_n : Constant  Value=CC.as_n_0
  c_sei : Sum  Inputs=+
  c_sei1 : Sum  Inputs=+
  ce_s : Sum
  del_sei : Sum
  del_sei1 : Constant  Value=CC.del_sei_init
  n selector : Selector  InputPortWidth=CC.n_nodes  IndexOptions=Index vector (dialog)  Indices=[1:CC.nn]  OutputSizes=1
  n+1 selector : Selector  InputPortWidth=CC.n_nodes  IndexOptions=Index vector (dialog)  Indices=[2:CC.nn+1]  OutputSizes=1
  wires:
  Exp/1 -> Gain6/1
  Divide1/1 -> Gain/1
  Gain/1 -> Exp/1
  eta_sr/1 -> Sum/2
  Usei/1 -> Sum/1
  Sum/1 -> Divide1/1
  Gain6/1 -> Product/1
  Product/1 -> To Workspace3/1, Gain7/1, c_sei1/1
  as_n/1 -> Product1/4
  del_sei/1 -> R Film/1, Product1/3
  Temp/1 -> Divide1/2
  Constant/1 -> Product1/2
  ce_s/1 -> Product/2
  n+1 selector/1 -> Sum1/2
  n selector/1 -> Sum1/1
  Sum1/1 -> c_sei/1
  Gain7/1 -> n selector/1, n+1 selector/1
  c_sei/1 -> Integrator/1
  Integrator/1 -> Gain1/1
  Gain1/1 -> del_sei/1
  del_sei1/1 -> del_sei/2
  c_sei1/1 -> Gain2/1
  Gain2/1 -> Product1/1
  Constant1/1 -> ce_s/2
  Constant2/1 -> ce_s/1
  Product1/1 -> Scope/1

== system SPM_trial_2_simulink/Plant/Electrolyte/Arrhenius ==
  Temp : Inport
  Constant : Constant  Value=1/CC.T
  Gain : Gain  Gain=CC.E_De/CC.R
  Math Function : Math
  Reciprocal : Product  Inputs=/
  Subtract : Sum  Inputs=+-
  Arr : Outport
  wires:
  Subtract/1 -> Gain/1
  Reciprocal/1 -> Subtract/2
  Constant/1 -> Subtract/1
  Math Function/1 -> Arr/1
  Temp/1 -> Reciprocal/1
  Gain/1 -> Math Function/1

== system SPM_trial_2_simulink/Plant/Electrolyte/Ce_ave_n ==
  dce : Inport
  ce_ave_p fcn : Fcn  Expr=u/(CC.nn+1)+CC.ce_init
  ce_n selector : Selector  InputPortWidth=CC.n_nodes  IndexOptions=Index vector (dialog)  Indices=[(np+ns)+1:(np+ns+nn)+1]  OutputSizes=1
  ce_n sum : Sum  Inputs=+
  ce_ave : Outport
  wires:
  ce_ave_p fcn/1 -> ce_ave/1
  dce/1 -> ce_n selector/1
  ce_n sum/1 -> ce_ave_p fcn/1
  ce_n selector/1 -> ce_n sum/1

== system SPM_trial_2_simulink/Plant/Electrolyte/Ce_ave_p ==
  dce : Inport
  ce_ave_p fcn : Fcn  Expr=u/(CC.np+1)+CC.ce_init
  ce_p selector : Selector  InputPortWidth=CC.n_nodes  IndexOptions=Index vector (dialog)  Indices=[1:CC.np+1]  OutputSizes=1
  ce_p sum : Sum  Inputs=+
  ce_ave : Outport
  wires:
  ce_ave_p fcn/1 -> ce_ave/1
  dce/1 -> ce_p selector/1
  ce_p sum/1 -> ce_ave_p fcn/1
  ce_p selector/1 -> ce_p sum/1

== system SPM_trial_2_simulink/Plant/Electrolyte Potential/Arrhenius ==
  Temp : Inport
  Constant : Constant  Value=1/CC.T
  Gain : Gain  Gain=CC.E_ke/CC.R
  Math Function : Math
  Reciprocal : Product  Inputs=/
  Subtract : Sum  Inputs=+-
  Arr : Outport
  wires:
  Subtract/1 -> Gain/1
  Reciprocal/1 -> Subtract/2
  Constant/1 -> Subtract/1
  Math Function/1 -> Arr/1
  Temp/1 -> Reciprocal/1
  Gain/1 -> Math Function/1

== system SPM_trial_2_simulink/Plant/Voltage/Arrhenius ==
  Temp : Inport
  Constant : Constant  Value=1/CC.T
  Gain : Gain  Gain=CC.E_r_p/CC.R
  Math Function : Math
  Reciprocal : Product  Inputs=/
  Subtract : Sum  Inputs=+-
  Arr : Outport
  wires:
  Subtract/1 -> Gain/1
  Reciprocal/1 -> Subtract/2
  Constant/1 -> Subtract/1
  Math Function/1 -> Arr/1
  Temp/1 -> Reciprocal/1
  Gain/1 -> Math Function/1

== system SPM_trial_2_simulink/Plant/Voltage/Arrhenius1 ==
  Temp : Inport
  Constant : Constant  Value=1/CC.T
  Gain : Gain  Gain=CC.E_r_n/CC.R
  Math Function : Math
  Reciprocal : Product  Inputs=/
  Subtract : Sum  Inputs=+-
  Arr : Outport
  wires:
  Subtract/1 -> Gain/1
  Reciprocal/1 -> Subtract/2
  Constant/1 -> Subtract/1
  Math Function/1 -> Arr/1
  Temp/1 -> Reciprocal/1
  Gain/1 -> Math Function/1

== system SPM_trial_2_simulink/Plant/Voltage/eta_p ==
  i0 : Inport
  j : Inport  Port=2
  Temp : Inport  Port=3
  Asinh : Trigonometry  Operator=asinh
  Fcn : Fcn  Expr=u(2)*CC.F/2/u(1)
  Gain : Gain  Gain=(CC.R/0.5/CC.F)
  Mux5 : Mux  Inputs=2
  Temp_mul : Product
  eta : Outport
  wires:
  Asinh/1 -> Temp_mul/2
  Fcn/1 -> Asinh/1
  i0/1 -> Mux5/1
  j/1 -> Mux5/2
  Mux5/1 -> Fcn/1
  Gain/1 -> eta/1
  Temp_mul/1 -> Gain/1
  Temp/1 -> Temp_mul/1

== system SPM_trial_2_simulink/Plant/Voltage/etan ==
  i0 : Inport
  j : Inport  Port=2
  Temp : Inport  Port=3
  Asinh : Trigonometry  Operator=asinh
  Fcn : Fcn  Expr=u(2)*CC.F/2/u(1)
  Gain : Gain  Gain=(CC.R/0.5/CC.F)
  Mux5 : Mux  Inputs=2
  Temp_mul : Product
  eta : Outport
  wires:
  Asinh/1 -> Temp_mul/2
  Fcn/1 -> Asinh/1
  i0/1 -> Mux5/1
  j/1 -> Mux5/2
  Mux5/1 -> Fcn/1
  Gain/1 -> eta/1
  Temp_mul/1 -> Gain/1
  Temp/1 -> Temp_mul/1

== system SPM_trial_2_simulink/Plant/Voltage/i0_n ==
  css : Inport
  ce_ave : Inport  Port=2
  Fcn : Fcn  Expr=u(2)*u(1)*(CC.cs_max_n-u(1))
  Gain : Gain  Gain=CC.k0_n.*CC.F
  Mux : Mux  Inputs=2
  Square Root : Sqrt
  i0 : Outport
  wires:
  Mux/1 -> Fcn/1
  ce_ave/1 -> Mux/2
  Square Root/1 -> Gain/1
  Gain/1 -> i0/1
  css/1 -> Mux/1
  Fcn/1 -> Square Root/1

== system SPM_trial_2_simulink/Plant/Voltage/i0_p ==
  css : Inport
  ce_ave : Inport  Port=2
  Fcn : Fcn  Expr=u(2)*u(1)*(CC.cs_max_p-u(1))
  Gain : Gain  Gain=CC.k0_p.*CC.F
  Mux : Mux  Inputs=2
  Square Root : Sqrt
  i0 : Outport
  wires:
  Mux/1 -> Fcn/1
  ce_ave/1 -> Mux/2
  Square Root/1 -> Gain/1
  Gain/1 -> i0/1
  css/1 -> Mux/1
  Fcn/1 -> Square Root/1

== matlab function SPM_trial_2_simulink/Plant/Voltage/Un ==
  data: u input; y output
function y = fcn(u)

y = Un_0(u);

== matlab function SPM_trial_2_simulink/Plant/Voltage/Up ==
  data: u input; y output
function y = fcn(u)

y = Up_1(u);

== matlab function SPM_trial_2_simulink/Plant/Expansion/expansion ==
  data: x1 input; up output; x2 input; nr input; Rp_0 input; Rn_0 input; un output
function [up,un] = fcn(x1,x2,nr,Rp_0,Rn_0)
Rvec_p = 0:Rp_0/nr:Rp_0;
cube_p = ((Rvec_p(2:end)).^3-(Rvec_p(1:end-1)).^3);
Rvec_n = 0:Rn_0/nr:Rn_0;
cube_n = ((Rvec_n(2:end)).^3-(Rvec_n(1:end-1)).^3);

Mp = arrayfun(@ep_1, x1');
up = ((cube_p.*(Mp(1:end-1)+Mp(2:end))/2)*ones(nr,1))/(Rp_0^2)/3;
Mn = arrayfun(@en, x2');
un = ((cube_n.*(Mn(1:end-1)+Mn(2:end))/2)*ones(nr,1))/(Rn_0^2)/3;

end

== matlab function SPM_trial_2_simulink/Plant/Cathode/cs_ave_p_obs ==
  data: cs_p input; csavg_p_obs output; nr input; Rp_0 input
function csavg_p_obs = fcn(cs_p,nr,Rp_0)
cs_p = cs_p';
Rvec = 0:Rp_0/nr:Rp_0;
cube = ((Rvec(2:end)).^3-(Rvec(1:end-1)).^3);
muln = (cs_p(1:end-1)+cs_p(2:end))/2;
csavg_p_obs = ((cube.*muln)*ones(nr,1))/(Rp_0^3);

== matlab function SPM_trial_2_simulink/Plant/Anode/cs_ave_n_obs ==
  data: cs_n input; csavg_n_obs output; nr input; Rn_0 input
function csavg_n_obs = fcn(cs_n,nr,Rn_0)
cs_n = cs_n';
Rvec = 0:Rn_0/nr:Rn_0;
cube = ((Rvec(2:end)).^3-(Rvec(1:end-1)).^3);
muln = (cs_n(1:end-1)+cs_n(2:end))/2;
csavg_n_obs = ((cube.*muln)*ones(nr,1))/(Rn_0^3);

== matlab function SPM_trial_2_simulink/Plant/Degradation/Mechanical Stress/sigma ==
  data: cs_n input; sigma_r output; nr input [0..nr+1]; Rn_0 input; const input; sigma_t output
function [sigma_r,sigma_t] = fcn(cs_n,nr,Rn_0,const) %,sigma_r,sigma_t
cs_n = cs_n';
Rvec = 0:Rn_0/nr:Rn_0;
cube = ((Rvec(2:end)).^3-(Rvec(1:end-1)).^3);
muln = (cs_n(1:end-1)+cs_n(2:end))/2;
% csavg_n = ((cube.*muln)*ones(nr,1))/(Rn_0^3);
% csavg_n_obs = ((cube.*muln)*ones(nr,1))/(Rn_0^3);

sigma_r = zeros(size(cs_n'));
sigma_r(1) = (2*const)*(1/Rn_0^3*(1/3*(cube.*muln)*ones(nr,1))-1/3*cs_n(1));
sigma_t = zeros(size(cs_n'));
sigma_t(1) = (1*const)*(2/Rn_0^3*(1/3*(cube.*muln)*ones(nr,1))+1/3*cs_n(1)-cs_n(1));
for i=1:nr
    sigma_r(i+1) = (2*const)*(1/Rn_0^3*(1/3*(cube.*muln)*ones(nr,1))-1/(i/nr*Rn_0)^3*(1/3*(cube(1:i).*muln(1:i))*ones(i,1)));
    sigma_t(i+1) = (1*const)*(2/Rn_0^3*(1/3*(cube.*muln)*ones(nr,1))+1/(i/nr*Rn_0)^3*(1/3*(cube(1:i).*muln(1:i))*ones(i,1))-cs_n(i+1));
end

end
